simulink model "SCo2"  (Simulink 8.5)
settings: Solver=ode23tb  SolverMode=SingleTasking  StartTime=0.0  StopTime=0.1  MaxStep=2e-4  RelTol=1e-3  AbsTol=1e-6
libraries: powerlib x100, powerlib_extras x21
(part 1 of 2)
settings Model: Creator=azadpour  LastModifiedBy=PC  ExtModeTrigMode=oneshot  ExtModeArmWhenConnect=off
settings DataIOCC: LimitDataPoints=off
settings OptimizationCC: BlockReduction=off  BooleanDataType=off  ExpressionDepthLimit=128  InitFltsAndDblsToZero=on
settings DebuggingCC: SaveWithParameterizedLinksMsg=none  SignalResolutionControl=TryResolveAllWithWarning  MultiTaskDSMMsg=warning  MultiTaskCondExecSysMsg=none  FcnCallInpInsideContextMsg=UseLocalSettings  StateNameClashWarn=none
settings HardwareCC: TargetUnknown=on
settings GRTTargetCC: TargetFcnLib=ansi_tfl_tmw.mat

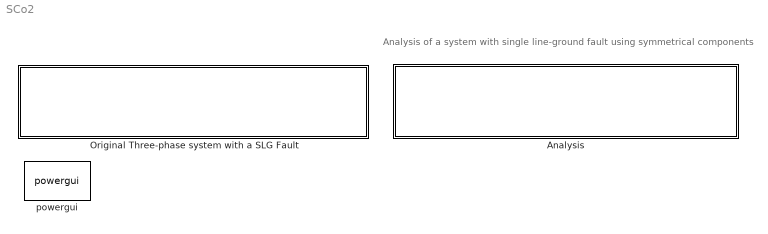
== system SCo2 ==
  note: Analysis of a system with single line-ground fault using symmetrical components
  Analysis : Subsystem
      mask init:
      | get_param('SCo2/Analysis/Fault Connection in Symmetrical Components','Name');
      mask Display: disp('Analysis of the system using Sequence Networks');
  Original Three-phase system with a SLG Fault : Subsystem
      mask Display: disp('Original Three-phase system with a SLG Fault')
  powergui : powerlib/powergui  Priority=1  SimulationMode=Continuous  SolverType=Tustin/Backward Euler (TBE)  SampleTime=50e-6  frequency=60  SPID=off  DisableSnubberDevices=off  DisableRonSwitches=off  DisableVfSwitches=off  SwTol=0  DisplayEquations=off  Interpol=off  methode=off  Ts=100  FunctionMessages=off  echomessages=off  HookPort=off  EnableUseOfTLC=off  x0status=blocks  frequencyindice=60  Pbase=100e6  ErrMax=1e-4  Iterations=50  UnitsV=kV  UnitsW=MW  buscounter=0  RestoreLinks=warning  ResistiveCurrentMeasurement=off  Frange=[0:2:500]  Ylog=off  Xlog=on  ShowGrid=off  save=off  variable=ZData  structure=0  ZoomFFT=off  StartTime=0.0  cycles=1  DisplayStyle=1  fundamental=60  FreqAxis=off  MaxFrequency=1000  frequencyindicesteady=1  RmsSteady=1  display=off

== system SCo2/Analysis ==
  note: Analysis using symmetrical networks
  Connected Symmetrical Networks : Subsystem
      mask Display: disp('Connected\n Sequence\n Networks')
  Fault Connection in Symmetrical Components : Subsystem
      mask Display: disp('Fault connection\n in\n symmetrical components')
  Negative Sequence Network : Subsystem
      mask Display: disp('Negative sequence network')
  Positive Sequence Network : Subsystem
      mask Display: disp('Positive sequence network')
  Zero Sequence Network : Subsystem
      mask Display: disp('Zero sequence network')

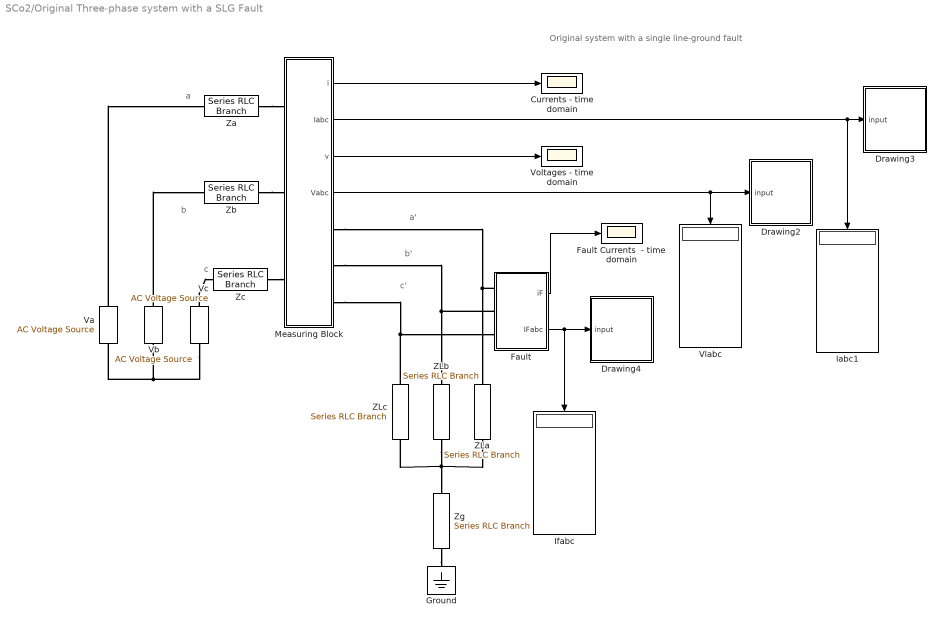
== system SCo2/Original Three-phase system with a SLG Fault ==
  note: a
  note: a'
  note: b
  note: b'
  note: c'
  note: c
  note: Original system with a single line-ground fault
  Currents - time domain : Scope
      settings: TickLabels=on
  Drawing2 : Subsystem  mask(ABC and 012 Phasor Display){Bactive=off}
      mask prompts: Bactive "Block active"
      mask init:
      | global count;
      | count=0;
      mask Display: disp('Display \nabc \nand \n012\nphasors');
  Drawing3 : Subsystem  mask(ABC and 012 Phasor Display){Bactive=off}
      mask prompts: Bactive "Block active"
      mask init:
      | global count;
      | count=0;
      mask Display: disp('Display \nabc \nand \n012\nphasors');
  Drawing4 : Subsystem  mask(ABC and 012 Phasor Display){Bactive=off}
      mask prompts: Bactive "Block active"
      mask init:
      | global count;
      | count=0;
      mask Display: disp('Display \nabc \nand \n012\nphasors');
  Fault : Subsystem
  Fault Currents  - time domain : Scope
      settings: TickLabels=on
  Ground : powerlib/Elements/Ground  LConnTagsString=a
  Iabc1 : Display
  Ifabc : Display
  Measuring Block : Subsystem
  Va : powerlib/Electrical Sources/AC Voltage Source  Amplitude=1  Phase=0  Frequency=60  SampleTime=0  Measurements=None
  Vb : powerlib/Electrical Sources/AC Voltage Source  Amplitude=1  Phase=-120  Frequency=60  SampleTime=0  Measurements=None
  Vc : powerlib/Electrical Sources/AC Voltage Source  Amplitude=1  Phase=120  Frequency=60  SampleTime=0  Measurements=None
  Vlabc : Display
  Voltages - time domain : Scope
      settings: TickLabels=on
  ZLa : powerlib/Elements/Series RLC Branch  LConnTagsString=__new0  RConnTagsString=__new0  BranchType=RL  Resistance=0.1736  Inductance=0.9848/(2*pi*60)  SetiL0=off  InitialCurrent=0  Capacitance=1.0  Setx0=off  InitialVoltage=0  Measurements=None
  ZLb : powerlib/Elements/Series RLC Branch  LConnTagsString=__new0  RConnTagsString=__new0  BranchType=RL  Resistance=0.1736  Inductance=0.9848/(2*pi*60)  SetiL0=off  InitialCurrent=0  Capacitance=1.0  Setx0=off  InitialVoltage=0  Measurements=None
  ZLc : powerlib/Elements/Series RLC Branch  LConnTagsString=__new0  RConnTagsString=__new0  BranchType=RL  Resistance=0.1736  Inductance=0.9848/(2*pi*60)  SetiL0=off  InitialCurrent=0  Capacitance=1.0  Setx0=off  InitialVoltage=0  Measurements=None
  Za : powerlib/Elements/Series RLC Branch  LConnTagsString=__new0  RConnTagsString=__new0  BranchType=RL  Resistance=0.0347  Inductance=0.1970/(2*pi*60)  SetiL0=off  InitialCurrent=0  Capacitance=1.0  Setx0=off  InitialVoltage=0  Measurements=None
  Zb : powerlib/Elements/Series RLC Branch  LConnTagsString=__new0  RConnTagsString=__new0  BranchType=RL  Resistance=0.0347  Inductance=0.1970/(2*pi*60)  SetiL0=off  InitialCurrent=0  Capacitance=1.0  Setx0=off  InitialVoltage=0  Measurements=None
  Zc : powerlib/Elements/Series RLC Branch  LConnTagsString=__new0  RConnTagsString=__new0  BranchType=RL  Resistance=0.0347  Inductance=0.1970/(2*pi*60)  SetiL0=off  InitialCurrent=0  Capacitance=1.0  Setx0=off  InitialVoltage=0  Measurements=None
  Zg : powerlib/Elements/Series RLC Branch  LConnTagsString=__new0  RConnTagsString=__new0  BranchType=RL  Resistance=0.0695  Inductance=0.3939/(2*pi*60)  SetiL0=off  InitialCurrent=0  Capacitance=1.0  Setx0=off  InitialVoltage=0  Measurements=None
  wires:
  Fault/1(iF) -> Fault Currents  - time domain/1
  Fault/2(IFabc) -> Drawing4/1(input), Ifabc/1
  Measuring Block/1(i) -> Currents - time domain/1
  Measuring Block/4(Vabc) -> Drawing2/1(input), Vlabc/1
  Measuring Block/3(v) -> Voltages - time domain/1
  Measuring Block/2(Iabc) -> Drawing3/1(input), Iabc1/1
  connections:
  Vc/LConn1 -- Va/LConn1 -- Vb/LConn1
  Va/RConn1 -- Za/LConn1
  Vc/RConn1 -- Zc/LConn1
  Za/RConn1 -- Measuring Block/LConn1
  Zc/RConn1 -- Measuring Block/LConn3
  Vb/RConn1 -- Zb/LConn1
  Zb/RConn1 -- Measuring Block/LConn2
  ZLc/LConn1 -- Fault/LConn3 -- Measuring Block/RConn3
  Fault/LConn2 -- ZLb/LConn1 -- Measuring Block/RConn2
  Fault/LConn1 -- ZLa/LConn1 -- Measuring Block/RConn1
  ZLa/RConn1 -- ZLc/RConn1 -- ZLb/RConn1 -- Zg/LConn1
  Zg/RConn1 -- Ground/LConn1

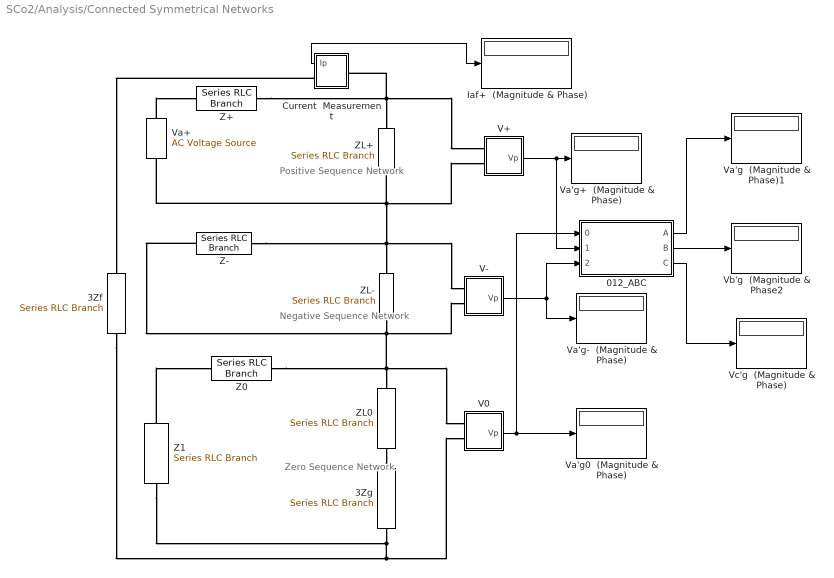
== system SCo2/Analysis/Connected Symmetrical Networks ==
  note: Positive Sequence Network
  note: Negative Sequence Network
  note: Zero Sequence Network
  012_ABC : Subsystem
      mask init:
      | a=cos(120*pi/180)+i*sin(120*pi/180);
      | A=[1 1 1; 1 a^2 a; 1 a a^2];
      mask Display: disp('012_ABC');
  3Zf : powerlib/Elements/Series RLC Branch  LConnTagsString=__new0  RConnTagsString=__new0  BranchType=RL  Resistance=3*0.0174  Inductance=3*0.0985/(2*pi*60)  SetiL0=off  InitialCurrent=0  Capacitance=1.0  Setx0=off  InitialVoltage=0  Measurements=None
  3Zg : powerlib/Elements/Series RLC Branch  LConnTagsString=__new0  RConnTagsString=__new0  BranchType=RL  Resistance=3*0.0695  Inductance=3*0.3939/(2*pi*60)  SetiL0=off  InitialCurrent=0  Capacitance=1.0  Setx0=off  InitialVoltage=0  Measurements=None
  Current  Measurement : Subsystem
  Iaf+  (Magnitude & Phase) : Display
  V+ : Subsystem
  V- : Subsystem
  V0 : Subsystem
  Va'g  (Magnitude & Phase)1 : Display
  Va'g+  (Magnitude & Phase) : Display
  Va'g-  (Magnitude & Phase) : Display
  Va'g0  (Magnitude & Phase) : Display
  Va+ : powerlib/Electrical Sources/AC Voltage Source  Amplitude=1  Phase=0  Frequency=60  SampleTime=0  Measurements=None
  Vb'g  (Magnitude & Phase2 : Display
  Vc'g  (Magnitude & Phase) : Display
  Z+ : powerlib/Elements/Series RLC Branch  LConnTagsString=__new0  RConnTagsString=__new0  BranchType=RL  Resistance=0.0347  Inductance=0.1970/(2*pi*60)  SetiL0=off  InitialCurrent=0  Capacitance=1.0  Setx0=off  InitialVoltage=0  Measurements=None
  Z- : powerlib/Elements/Series RLC Branch  LConnTagsString=__new0  RConnTagsString=__new0  BranchType=RL  Resistance=0.0347  Inductance=0.1970/(2*pi*60)  SetiL0=off  InitialCurrent=0  Capacitance=1.0  Setx0=off  InitialVoltage=0  Measurements=None
  Z0 : powerlib/Elements/Series RLC Branch  LConnTagsString=__new0  RConnTagsString=__new0  BranchType=RL  Resistance=0.0347  Inductance=0.1970/(2*pi*60)  SetiL0=off  InitialCurrent=0  Capacitance=1.0  Setx0=off  InitialVoltage=0  Measurements=None
  Z1 : powerlib/Elements/Series RLC Branch  LConnTagsString=__new0  RConnTagsString=__new0  BranchType=Open circuit  Resistance=1  Inductance=1.0  SetiL0=off  InitialCurrent=0  Capacitance=1.0  Setx0=off  InitialVoltage=0  Measurements=None
  ZL+ : powerlib/Elements/Series RLC Branch  LConnTagsString=__new0  RConnTagsString=__new0  BranchType=RL  Resistance=0.1736  Inductance=0.9848/(2*pi*60)  SetiL0=off  InitialCurrent=0  Capacitance=1.0  Setx0=off  InitialVoltage=0  Measurements=None
  ZL- : powerlib/Elements/Series RLC Branch  LConnTagsString=__new0  RConnTagsString=__new0  BranchType=RL  Resistance=0.1736  Inductance=0.9848/(2*pi*60)  SetiL0=off  InitialCurrent=0  Capacitance=1.0  Setx0=off  InitialVoltage=0  Measurements=None
  ZL0 : powerlib/Elements/Series RLC Branch  LConnTagsString=__new0  RConnTagsString=__new0  BranchType=RL  Resistance=0.1736  Inductance=0.9848/(2*pi*60)  SetiL0=off  InitialCurrent=0  Capacitance=1.0  Setx0=off  InitialVoltage=0  Measurements=None
  wires:
  Current  Measurement/1(Ip) -> Iaf+  (Magnitude & Phase)/1
  012_ABC/1(A) -> Va'g  (Magnitude & Phase)1/1
  012_ABC/2(B) -> Vb'g  (Magnitude & Phase2/1
  012_ABC/3(C) -> Vc'g  (Magnitude & Phase)/1
  V0/1(Vp) -> Va'g0  (Magnitude & Phase)/1, 012_ABC/1(0)
  V+/1(Vp) -> Va'g+  (Magnitude & Phase)/1, 012_ABC/2(1)
  V-/1(Vp) -> Va'g-  (Magnitude & Phase)/1, 012_ABC/3(2)
  connections:
  Z1/RConn1 -- 3Zf/RConn1 -- V0/LConn2 -- 3Zg/RConn1
  Va+/RConn1 -- Z+/LConn1
  V-/LConn1 -- ZL-/LConn1 -- Z-/RConn1 -- Va+/LConn1 -- V+/LConn2 -- ZL+/RConn1
  Z+/RConn1 -- V+/LConn1 -- ZL+/LConn1 -- Current  Measurement/LConn1
  Current  Measurement/RConn1 -- 3Zf/LConn1
  Z0/RConn1 -- V-/LConn2 -- ZL-/RConn1 -- Z-/LConn1 -- ZL0/LConn1 -- V0/LConn1
  Z1/LConn1 -- Z0/LConn1
  ZL0/RConn1 -- 3Zg/LConn1

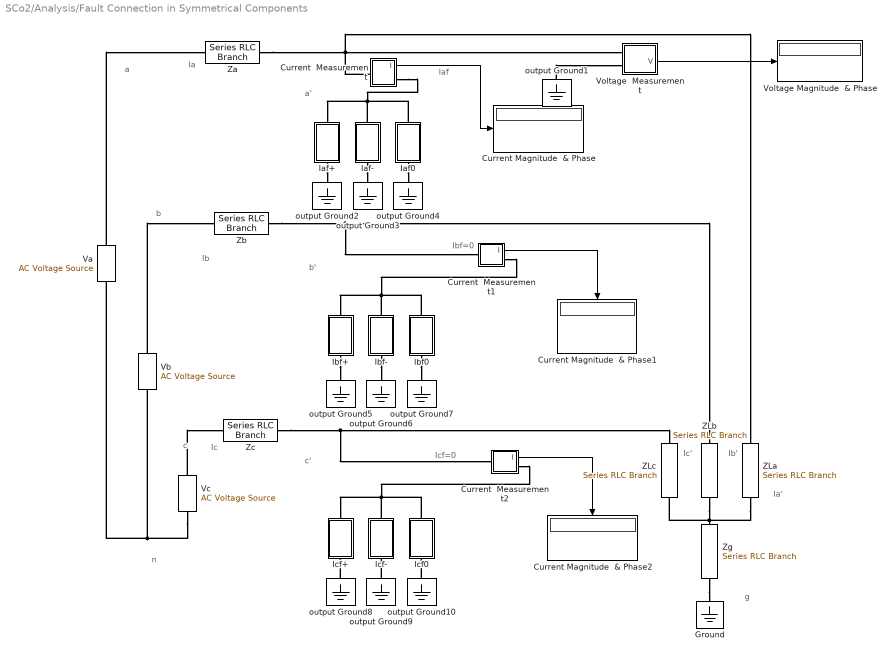
== system SCo2/Analysis/Fault Connection in Symmetrical Components ==
  note: Ibf=0
  note: Icf=0
  note: Ia
  note: Ib
  note: Ic
  note: Ia'
  note: Ib'
  note: Ic'
  note: a
  note: b
  note: c
  note: c'
  note: b'
  note: a'
  note: Iaf
  note: g
  note: n
  Current  Measurement : Subsystem
  Current  Measurement1 : Subsystem
  Current  Measurement2 : Subsystem
  Current Magnitude  & Phase : Display
  Current Magnitude  & Phase1 : Display
  Current Magnitude  & Phase2 : Display
  Ground : powerlib/Elements/Ground  LConnTagsString=a
  Iaf+ : Subsystem  mask{A=-0.8823/3, P=-80, F=60}
      mask prompts: A "Peak amplitude(A)"; P "Phase (deg)"; F "Freqiuency"
      mask Display: plot(-50,-35,50,50-15,[0,9,18,24,29,30,29,24,18,9,0,-9,-18,-24,-29,-30,-29,-24,-18,-9,0],[30,29,24,18,9,0,-9,-18,-24,-29,-30,-29,-24,-18,-9,0,9,18,24,29,30],[-20 5 5 20 5 5],[2 2 12 2 -8 2],[-50 -30],[0 0],[50,30],[0 0],[45 35 40 40 40],[15 15 15 20 10]);
  Iaf- : Subsystem  mask{A=-0.8823/3, P=-80, F=60}
      mask prompts: A "Peak amplitude(A)"; P "Phase (deg)"; F "Freqiuency"
      mask Display: plot(-50,-35,50,50-15,[0,9,18,24,29,30,29,24,18,9,0,-9,-18,-24,-29,-30,-29,-24,-18,-9,0],[30,29,24,18,9,0,-9,-18,-24,-29,-30,-29,-24,-18,-9,0,9,18,24,29,30],[-20 5 5 20 5 5],[2 2 12 2 -8 2],[-50 -30],[0 0],[50,30],[0 0],[45 35 40 40 40],[15 15 15 20 10]);
  Iaf0 : Subsystem  mask{A=-0.8823/3, P=-80, F=60}
      mask prompts: A "Peak amplitude(A)"; P "Phase (deg)"; F "Freqiuency"
      mask Display: plot(-50,-35,50,50-15,[0,9,18,24,29,30,29,24,18,9,0,-9,-18,-24,-29,-30,-29,-24,-18,-9,0],[30,29,24,18,9,0,-9,-18,-24,-29,-30,-29,-24,-18,-9,0,9,18,24,29,30],[-20 5 5 20 5 5],[2 2 12 2 -8 2],[-50 -30],[0 0],[50,30],[0 0],[45 35 40 40 40],[15 15 15 20 10]);
  Ibf+ : Subsystem  mask{A=-0.8823/3, P=-80-120, F=60}
      mask prompts: A "Peak amplitude(A)"; P "Phase (deg)"; F "Freqiuency"
      mask Display: plot(-50,-35,50,50-15,[0,9,18,24,29,30,29,24,18,9,0,-9,-18,-24,-29,-30,-29,-24,-18,-9,0],[30,29,24,18,9,0,-9,-18,-24,-29,-30,-29,-24,-18,-9,0,9,18,24,29,30],[-20 5 5 20 5 5],[2 2 12 2 -8 2],[-50 -30],[0 0],[50,30],[0 0],[45 35 40 40 40],[15 15 15 20 10]);
  Ibf- : Subsystem  mask{A=-0.8823/3, P=-80+120, F=60}
      mask prompts: A "Peak amplitude(A)"; P "Phase (deg)"; F "Freqiuency"
      mask Display: plot(-50,-35,50,50-15,[0,9,18,24,29,30,29,24,18,9,0,-9,-18,-24,-29,-30,-29,-24,-18,-9,0],[30,29,24,18,9,0,-9,-18,-24,-29,-30,-29,-24,-18,-9,0,9,18,24,29,30],[-20 5 5 20 5 5],[2 2 12 2 -8 2],[-50 -30],[0 0],[50,30],[0 0],[45 35 40 40 40],[15 15 15 20 10]);
  Ibf0 : Subsystem  mask{A=-0.8823/3, P=-80, F=60}
      mask prompts: A "Peak amplitude(A)"; P "Phase (deg)"; F "Freqiuency"
      mask Display: plot(-50,-35,50,50-15,[0,9,18,24,29,30,29,24,18,9,0,-9,-18,-24,-29,-30,-29,-24,-18,-9,0],[30,29,24,18,9,0,-9,-18,-24,-29,-30,-29,-24,-18,-9,0,9,18,24,29,30],[-20 5 5 20 5 5],[2 2 12 2 -8 2],[-50 -30],[0 0],[50,30],[0 0],[45 35 40 40 40],[15 15 15 20 10]);
  Icf+ : Subsystem  mask{A=-0.8823/3, P=-80+120, F=60}
      mask prompts: A "Peak amplitude(A)"; P "Phase (deg)"; F "Freqiuency"
      mask Display: plot(-50,-35,50,50-15,[0,9,18,24,29,30,29,24,18,9,0,-9,-18,-24,-29,-30,-29,-24,-18,-9,0],[30,29,24,18,9,0,-9,-18,-24,-29,-30,-29,-24,-18,-9,0,9,18,24,29,30],[-20 5 5 20 5 5],[2 2 12 2 -8 2],[-50 -30],[0 0],[50,30],[0 0],[45 35 40 40 40],[15 15 15 20 10]);
  Icf- : Subsystem  mask{A=-0.8823/3, P=-80-120, F=60}
      mask prompts: A "Peak amplitude(A)"; P "Phase (deg)"; F "Freqiuency"
      mask Display: plot(-50,-35,50,50-15,[0,9,18,24,29,30,29,24,18,9,0,-9,-18,-24,-29,-30,-29,-24,-18,-9,0],[30,29,24,18,9,0,-9,-18,-24,-29,-30,-29,-24,-18,-9,0,9,18,24,29,30],[-20 5 5 20 5 5],[2 2 12 2 -8 2],[-50 -30],[0 0],[50,30],[0 0],[45 35 40 40 40],[15 15 15 20 10]);
  Icf0 : Subsystem  mask{A=-0.8823/3, P=-80, F=60}
      mask prompts: A "Peak amplitude(A)"; P "Phase (deg)"; F "Freqiuency"
      mask Display: plot(-50,-35,50,50-15,[0,9,18,24,29,30,29,24,18,9,0,-9,-18,-24,-29,-30,-29,-24,-18,-9,0],[30,29,24,18,9,0,-9,-18,-24,-29,-30,-29,-24,-18,-9,0,9,18,24,29,30],[-20 5 5 20 5 5],[2 2 12 2 -8 2],[-50 -30],[0 0],[50,30],[0 0],[45 35 40 40 40],[15 15 15 20 10]);
  Va : powerlib/Electrical Sources/AC Voltage Source  Amplitude=1  Phase=0  Frequency=60  SampleTime=0  Measurements=None
  Vb : powerlib/Electrical Sources/AC Voltage Source  Amplitude=1  Phase=-120  Frequency=60  SampleTime=0  Measurements=None
  Vc : powerlib/Electrical Sources/AC Voltage Source  Amplitude=1  Phase=120  Frequency=60  SampleTime=0  Measurements=None
  Voltage  Measurement : Subsystem
  Voltage Magnitude  & Phase : Display
  ZLa : powerlib/Elements/Series RLC Branch  LConnTagsString=__new0  RConnTagsString=__new0  BranchType=RL  Resistance=0.1736  Inductance=0.9848/(2*pi*60)  SetiL0=off  InitialCurrent=0  Capacitance=1.0  Setx0=off  InitialVoltage=0  Measurements=None
  ZLb : powerlib/Elements/Series RLC Branch  LConnTagsString=__new0  RConnTagsString=__new0  BranchType=RL  Resistance=0.1736  Inductance=0.9848/(2*pi*60)  SetiL0=off  InitialCurrent=0  Capacitance=1.0  Setx0=off  InitialVoltage=0  Measurements=None
  ZLc : powerlib/Elements/Series RLC Branch  LConnTagsString=__new0  RConnTagsString=__new0  BranchType=RL  Resistance=0.1736  Inductance=0.9848/(2*pi*60)  SetiL0=off  InitialCurrent=0  Capacitance=1.0  Setx0=off  InitialVoltage=0  Measurements=None
  Za : powerlib/Elements/Series RLC Branch  LConnTagsString=__new0  RConnTagsString=__new0  BranchType=RL  Resistance=0.0347  Inductance=0.1970/(2*pi*60)  SetiL0=off  InitialCurrent=0  Capacitance=1.0  Setx0=off  InitialVoltage=0  Measurements=None
  Zb : powerlib/Elements/Series RLC Branch  LConnTagsString=__new0  RConnTagsString=__new0  BranchType=RL  Resistance=0.0347  Inductance=0.1970/(2*pi*60)  SetiL0=off  InitialCurrent=0  Capacitance=1.0  Setx0=off  InitialVoltage=0  Measurements=None
  Zc : powerlib/Elements/Series RLC Branch  LConnTagsString=__new0  RConnTagsString=__new0  BranchType=RL  Resistance=0.0347  Inductance=0.1970/(2*pi*60)  SetiL0=off  InitialCurrent=0  Capacitance=1.0  Setx0=off  InitialVoltage=0  Measurements=None
  Zg : powerlib/Elements/Series RLC Branch  LConnTagsString=__new0  RConnTagsString=__new0  BranchType=RL  Resistance=0.0695  Inductance=0.3939/(2*pi*60)  SetiL0=off  InitialCurrent=0  Capacitance=1.0  Setx0=off  InitialVoltage=0  Measurements=None
  output Ground{1..10} (10 alike) : powerlib/Elements/Ground  LConnTagsString=a
  wires:
  Current  Measurement/1(I) -> Current Magnitude  & Phase/1
  Current  Measurement2/1(I) -> Current Magnitude  & Phase2/1
  Voltage  Measurement/1(V) -> Voltage Magnitude  & Phase/1
  Current  Measurement1/1(I) -> Current Magnitude  & Phase1/1
  connections:
  Va/RConn1 -- Za/LConn1
  output Ground1/LConn1 -- Voltage  Measurement/LConn2
  Vb/RConn1 -- Zb/LConn1
  Vc/RConn1 -- Zc/LConn1
  Zc/RConn1 -- ZLc/LConn1 -- Current  Measurement2/LConn1
  Zg/RConn1 -- Ground/LConn1
  Ibf+/LConn1 -- output Ground5/LConn1
  Ibf-/LConn1 -- output Ground6/LConn1
  Ibf0/LConn1 -- output Ground7/LConn1
  Ibf0/RConn1 -- Ibf+/RConn1 -- Ibf-/RConn1 -- Current  Measurement1/RConn1
  output Ground8/LConn1 -- Icf+/LConn1
  output Ground9/LConn1 -- Icf-/LConn1
  output Ground10/LConn1 -- Icf0/LConn1
  Icf0/RConn1 -- Icf+/RConn1 -- Icf-/RConn1 -- Current  Measurement2/RConn1
  ZLa/RConn1 -- ZLb/RConn1 -- Zg/LConn1 -- ZLc/RConn1
  Iaf0/RConn1 -- Iaf+/RConn1 -- Iaf-/RConn1 -- Current  Measurement/RConn1
  Iaf+/LConn1 -- output Ground2/LConn1
  Iaf-/LConn1 -- output Ground3/LConn1
  Iaf0/LConn1 -- output Ground4/LConn1
  Vc/LConn1 -- Va/LConn1 -- Vb/LConn1
  Current  Measurement/LConn1 -- Voltage  Measurement/LConn1 -- ZLa/LConn1 -- Za/RConn1
  Zb/RConn1 -- ZLb/LConn1 -- Current  Measurement1/LConn1

== system SCo2/Analysis/Negative Sequence Network ==
  Current  Measurement : Subsystem
  Iaf- : Subsystem  mask{A=-0.8823/3, P=-80, F=60}
      mask prompts: A "Peak amplitude(A)"; P "Phase (deg)"; F "Freqiuency"
      mask Display: plot(-50,-35,50,50-15,[0,9,18,24,29,30,29,24,18,9,0,-9,-18,-24,-29,-30,-29,-24,-18,-9,0],[30,29,24,18,9,0,-9,-18,-24,-29,-30,-29,-24,-18,-9,0,9,18,24,29,30],[-20 5 5 20 5 5],[2 2 12 2 -8 2],[-50 -30],[0 0],[50,30],[0 0],[45 35 40 40 40],[15 15 15 20 10]);
  Iaf- (Magnitude & Phase) : Display
  V- : Subsystem
  Va'g- (Magnitude & Phase) : Display
  ZLa : powerlib/Elements/Series RLC Branch  LConnTagsString=__new0  RConnTagsString=__new0  BranchType=RL  Resistance=0.1736  Inductance=0.9848/(2*pi*60)  SetiL0=off  InitialCurrent=0  Capacitance=1.0  Setx0=off  InitialVoltage=0  Measurements=None
  Za : powerlib/Elements/Series RLC Branch  LConnTagsString=__new0  RConnTagsString=__new0  BranchType=RL  Resistance=0.0347  Inductance=0.1970/(2*pi*60)  SetiL0=off  InitialCurrent=0  Capacitance=1.0  Setx0=off  InitialVoltage=0  Measurements=None
  wires:
  Current  Measurement/1(I) -> Iaf- (Magnitude & Phase)/1
  V-/1(V) -> Va'g- (Magnitude & Phase)/1
  connections:
  Za/RConn1 -- ZLa/LConn1 -- V-/LConn1 -- Current  Measurement/LConn1
  ZLa/RConn1 -- V-/LConn2 -- Za/LConn1 -- Iaf-/LConn1
  Current  Measurement/RConn1 -- Iaf-/RConn1

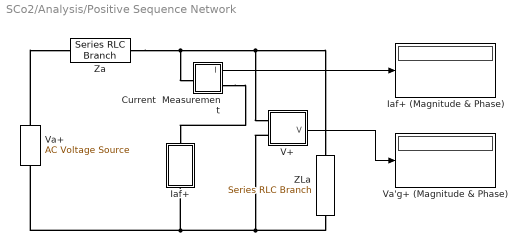
== system SCo2/Analysis/Positive Sequence Network ==
  Current  Measurement : Subsystem
  Iaf+ : Subsystem  mask{A=-0.8823/3, P=-80, F=60}
      mask prompts: A "Peak amplitude(A)"; P "Phase (deg)"; F "Freqiuency"
      mask Display: plot(-50,-35,50,50-15,[0,9,18,24,29,30,29,24,18,9,0,-9,-18,-24,-29,-30,-29,-24,-18,-9,0],[30,29,24,18,9,0,-9,-18,-24,-29,-30,-29,-24,-18,-9,0,9,18,24,29,30],[-20 5 5 20 5 5],[2 2 12 2 -8 2],[-50 -30],[0 0],[50,30],[0 0],[45 35 40 40 40],[15 15 15 20 10]);
  Iaf+ (Magnitude & Phase) : Display
  V+ : Subsystem
  Va'g+ (Magnitude & Phase) : Display
  Va+ : powerlib/Electrical Sources/AC Voltage Source  Amplitude=1  Phase=0  Frequency=60  SampleTime=0  Measurements=None
  ZLa : powerlib/Elements/Series RLC Branch  LConnTagsString=__new0  RConnTagsString=__new0  BranchType=RL  Resistance=0.1736  Inductance=0.9848/(2*pi*60)  SetiL0=off  InitialCurrent=0  Capacitance=1.0  Setx0=off  InitialVoltage=0  Measurements=None
  Za : powerlib/Elements/Series RLC Branch  LConnTagsString=__new0  RConnTagsString=__new0  BranchType=RL  Resistance=0.0347  Inductance=0.1970/(2*pi*60)  SetiL0=off  InitialCurrent=0  Capacitance=1.0  Setx0=off  InitialVoltage=0  Measurements=None
  wires:
  Current  Measurement/1(I) -> Iaf+ (Magnitude & Phase)/1
  V+/1(V) -> Va'g+ (Magnitude & Phase)/1
  connections:
  Va+/RConn1 -- Za/LConn1
  Za/RConn1 -- Current  Measurement/LConn1 -- ZLa/LConn1 -- V+/LConn1
  V+/LConn2 -- ZLa/RConn1 -- Iaf+/LConn1 -- Va+/LConn1
  Current  Measurement/RConn1 -- Iaf+/RConn1

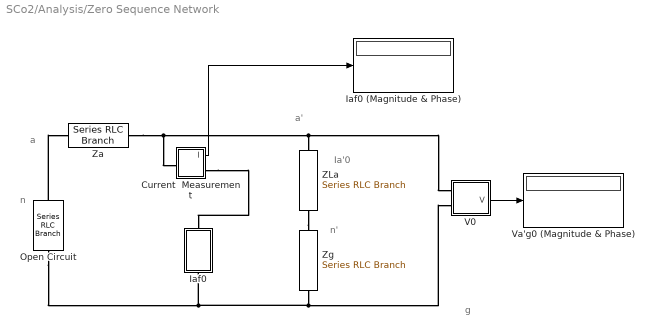
== system SCo2/Analysis/Zero Sequence Network ==
  note: n'
  note: n
  note: a
  note: a'
  note: g
  note: Ia'0
  Current  Measurement : Subsystem
  Iaf0 : Subsystem  mask{A=-0.8823/3, P=-80, F=60}
      mask prompts: A "Peak amplitude(A)"; P "Phase (deg)"; F "Freqiuency"
      mask Display: plot(-50,-35,50,50-15,[0,9,18,24,29,30,29,24,18,9,0,-9,-18,-24,-29,-30,-29,-24,-18,-9,0],[30,29,24,18,9,0,-9,-18,-24,-29,-30,-29,-24,-18,-9,0,9,18,24,29,30],[-20 5 5 20 5 5],[2 2 12 2 -8 2],[-50 -30],[0 0],[50,30],[0 0],[45 35 40 40 40],[15 15 15 20 10]);
  Iaf0 (Magnitude & Phase) : Display
  Open Circuit : powerlib/Elements/Series RLC Branch  LConnTagsString=__new0  RConnTagsString=__new0  BranchType=Open circuit  Resistance=1  Inductance=1e-3  SetiL0=off  InitialCurrent=0  Capacitance=1e-6  Setx0=off  InitialVoltage=0  Measurements=None
  V0 : Subsystem
  Va'g0 (Magnitude & Phase) : Display
  ZLa : powerlib/Elements/Series RLC Branch  LConnTagsString=__new0  RConnTagsString=__new0  BranchType=RL  Resistance=0.1736  Inductance=0.9848/(2*pi*60)  SetiL0=off  InitialCurrent=0  Capacitance=1.0  Setx0=off  InitialVoltage=0  Measurements=None
  Za : powerlib/Elements/Series RLC Branch  LConnTagsString=__new0  RConnTagsString=__new0  BranchType=RL  Resistance=0.0347  Inductance=0.1970/(2*pi*60)  SetiL0=off  InitialCurrent=0  Capacitance=1.0  Setx0=off  InitialVoltage=0  Measurements=None
  Zg : powerlib/Elements/Series RLC Branch  LConnTagsString=__new0  RConnTagsString=__new0  BranchType=RL  Resistance=3*0.0695  Inductance=3*0.3939/(2*pi*60)  SetiL0=off  InitialCurrent=0  Capacitance=1.0  Setx0=off  InitialVoltage=0  Measurements=None
  wires:
  Current  Measurement/1(I) -> Iaf0 (Magnitude & Phase)/1
  V0/1(V) -> Va'g0 (Magnitude & Phase)/1
  connections:
  Za/RConn1 -- ZLa/LConn1 -- V0/LConn1 -- Current  Measurement/LConn1
  Zg/RConn1 -- V0/LConn2 -- Open Circuit/RConn1 -- Iaf0/LConn1
  ZLa/RConn1 -- Zg/LConn1
  Current  Measurement/RConn1 -- Iaf0/RConn1
  Open Circuit/LConn1 -- Za/LConn1

== system SCo2/Original Three-phase system with a SLG Fault/Drawing2 ==
  input : Inport
  S-Function : S-Function  FunctionName=phdraw1c  Parameters=Bactive
  wires:
  input/1 -> S-Function/1

== system SCo2/Original Three-phase system with a SLG Fault/Drawing3 ==
  input : Inport
  S-Function : S-Function  FunctionName=phdraw1c  Parameters=Bactive
  wires:
  input/1 -> S-Function/1

== system SCo2/Original Three-phase system with a SLG Fault/Drawing4 ==
  input : Inport
  S-Function : S-Function  FunctionName=phdraw1c  Parameters=Bactive
  wires:
  input/1 -> S-Function/1

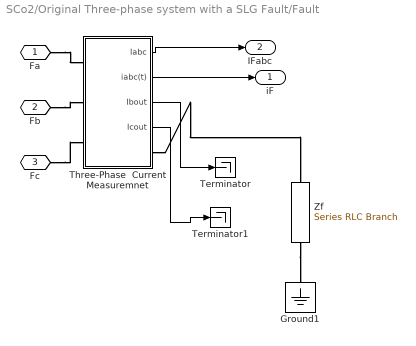
== system SCo2/Original Three-phase system with a SLG Fault/Fault ==
  Ground1 : powerlib/Elements/Ground  LConnTagsString=a
  Terminator : Terminator
  Terminator1 : Terminator
  Three-Phase  Current Measuremnet : Subsystem
  Zf : powerlib/Elements/Series RLC Branch  LConnTagsString=__new0  RConnTagsString=__new0  BranchType=RL  Resistance=0.0174  Inductance=0.0985/(2*pi*60)  SetiL0=off  InitialCurrent=0  Capacitance=1.0  Setx0=off  InitialVoltage=0  Measurements=None
  Fa : PMIOPort  Port=1  Side=Left
  Fb : PMIOPort  Port=2  Side=Left
  Fc : PMIOPort  Port=3  Side=Left
  iF : Outport
  IFabc : Outport  Port=2
  wires:
  Three-Phase  Current Measuremnet/1(Iabc) -> IFabc/1
  Three-Phase  Current Measuremnet/3(Ibout) -> Terminator/1
  Three-Phase  Current Measuremnet/4(Icout) -> Terminator1/1
  Three-Phase  Current Measuremnet/2(iabc(t)) -> iF/1
  connections:
  Three-Phase  Current Measuremnet/RConn1 -- Zf/LConn1
  Zf/RConn1 -- Ground1/LConn1
  Fb/RConn1 -- Three-Phase  Current Measuremnet/LConn2
  Fc/RConn1 -- Three-Phase  Current Measuremnet/LConn3
  Fa/RConn1 -- Three-Phase  Current Measuremnet/LConn1

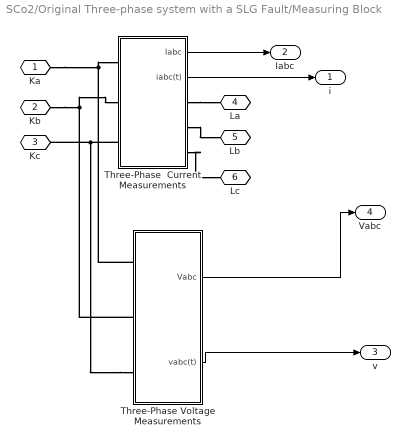
== system SCo2/Original Three-phase system with a SLG Fault/Measuring Block ==
  Three-Phase Voltage Measurements : Subsystem
  Three-Phase  Current Measurements : Subsystem
  Ka : PMIOPort  Port=1  Side=Left
  Kb : PMIOPort  Port=2  Side=Left
  Kc : PMIOPort  Port=3  Side=Left
  La : PMIOPort  Port=4  Side=Right
  Lb : PMIOPort  Port=5  Side=Right
  Lc : PMIOPort  Port=6  Side=Right
  i : Outport
  Iabc : Outport  Port=2
  v : Outport  Port=3
  Vabc : Outport  Port=4
  wires:
  Three-Phase  Current Measurements/1(Iabc) -> Iabc/1
  Three-Phase Voltage Measurements/1(Vabc) -> Vabc/1
  Three-Phase  Current Measurements/2(iabc(t)) -> i/1
  Three-Phase Voltage Measurements/2(vabc(t)) -> v/1
  connections:
  Three-Phase Voltage Measurements/LConn1 -- Ka/RConn1 -- Three-Phase  Current Measurements/LConn1
  Three-Phase Voltage Measurements/LConn2 -- Kb/RConn1 -- Three-Phase  Current Measurements/LConn2
  Three-Phase Voltage Measurements/LConn3 -- Kc/RConn1 -- Three-Phase  Current Measurements/LConn3
  Three-Phase  Current Measurements/RConn3 -- Lc/RConn1
  Three-Phase  Current Measurements/RConn2 -- Lb/RConn1
  Three-Phase  Current Measurements/RConn1 -- La/RConn1

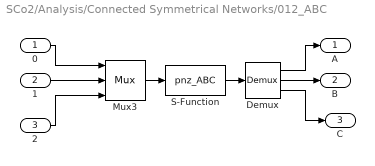
== system SCo2/Analysis/Connected Symmetrical Networks/012_ABC ==
  0 : Inport
  1 : Inport  Port=2
  2 : Inport  Port=3
  Demux : Demux  Outputs=3
  Mux3 : Mux  Inputs=3
  S-Function : S-Function  FunctionName=pnz_ABC  Parameters=A
  A : Outport  InitialOutput=0
  B : Outport  Port=2  InitialOutput=0
  C : Outport  Port=3  InitialOutput=0
  wires:
  Mux3/1 -> S-Function/1
  0/1 -> Mux3/1
  1/1 -> Mux3/2
  2/1 -> Mux3/3
  S-Function/1 -> Demux/1
  Demux/1 -> A/1
  Demux/2 -> B/1
  Demux/3 -> C/1

== system SCo2/Analysis/Connected Symmetrical Networks/Current  Measurement ==
  Current Measurement1 : powerlib/Measurements/Current Measurement  PhasorSimulation=off  OutputType=Magnitude  PSBequivalent=0
  Fourier1 : powerlib_extras/Measurements/Fourier  f1=60  n=1
  Mux1 : Mux  Inputs=2
  + : PMIOPort  Port=1  Side=Left
  - : PMIOPort  Port=2  Side=Right
  Ip : Outport  InitialOutput=0
  wires:
  Fourier1/2 -> Mux1/2
  Fourier1/1 -> Mux1/1
  Mux1/1 -> Ip/1
  Current Measurement1/1 -> Fourier1/1
  connections:
  +/RConn1 -- Current Measurement1/LConn1
  Current Measurement1/RConn1 -- -/RConn1

== system SCo2/Analysis/Connected Symmetrical Networks/V+ ==
  Fourier2 : powerlib_extras/Measurements/Fourier  f1=60  n=1
  Mux3 : Mux  Inputs=2
  Voltage Measurement1 : powerlib/Measurements/Voltage Measurement  PhasorSimulation=off  OutputType=Magnitude  PSBequivalent=0
  + : PMIOPort  Port=1  Side=Left
  - : PMIOPort  Port=2  Side=Left
  Vp : Outport  InitialOutput=0
  wires:
  Fourier2/1 -> Mux3/1
  Fourier2/2 -> Mux3/2
  Mux3/1 -> Vp/1
  Voltage Measurement1/1 -> Fourier2/1
  connections:
  +/RConn1 -- Voltage Measurement1/LConn1
  -/RConn1 -- Voltage Measurement1/LConn2

== system SCo2/Analysis/Connected Symmetrical Networks/V- ==
  Fourier2 : powerlib_extras/Measurements/Fourier  f1=60  n=1
  Mux3 : Mux  Inputs=2
  Voltage Measurement1 : powerlib/Measurements/Voltage Measurement  PhasorSimulation=off  OutputType=Magnitude  PSBequivalent=0
  + : PMIOPort  Port=1  Side=Left
  - : PMIOPort  Port=2  Side=Left
  Vp : Outport  InitialOutput=0
  wires:
  Fourier2/1 -> Mux3/1
  Fourier2/2 -> Mux3/2
  Mux3/1 -> Vp/1
  Voltage Measurement1/1 -> Fourier2/1
  connections:
  +/RConn1 -- Voltage Measurement1/LConn1
  -/RConn1 -- Voltage Measurement1/LConn2

== system SCo2/Analysis/Connected Symmetrical Networks/V0 ==
  Fourier2 : powerlib_extras/Measurements/Fourier  f1=60  n=1
  Mux3 : Mux  Inputs=2
  Voltage Measurement1 : powerlib/Measurements/Voltage Measurement  PhasorSimulation=off  OutputType=Magnitude  PSBequivalent=0
  + : PMIOPort  Port=1  Side=Left
  - : PMIOPort  Port=2  Side=Left
  Vp : Outport  InitialOutput=0
  wires:
  Mux3/1 -> Vp/1
  Fourier2/2 -> Mux3/2
  Fourier2/1 -> Mux3/1
  Voltage Measurement1/1 -> Fourier2/1
  connections:
  -/RConn1 -- Voltage Measurement1/LConn2
  +/RConn1 -- Voltage Measurement1/LConn1

== system SCo2/Analysis/Fault Connection in Symmetrical Components/Current  Measurement ==
  Current Magnitude  & Phase1 : Display
  Current Measurement1 : powerlib/Measurements/Current Measurement  PhasorSimulation=off  OutputType=Magnitude  PSBequivalent=0
  Fourier1 : powerlib_extras/Measurements/Fourier  f1=60  n=1
  Mux1 : Mux  Inputs=2
  + : PMIOPort  Port=1  Side=Left
  - : PMIOPort  Port=2  Side=Right
  I : Outport  InitialOutput=0
  wires:
  Fourier1/2 -> Mux1/2
  Fourier1/1 -> Mux1/1
  Mux1/1 -> I/1
  Current Measurement1/1 -> Fourier1/1, Current Magnitude  & Phase1/1
  connections:
  +/RConn1 -- Current Measurement1/LConn1
  Current Measurement1/RConn1 -- -/RConn1

== system SCo2/Analysis/Fault Connection in Symmetrical Components/Current  Measurement1 ==
  Current Magnitude  & Phase1 : Display
  Current Measurement1 : powerlib/Measurements/Current Measurement  PhasorSimulation=off  OutputType=Magnitude  PSBequivalent=0
  Fourier1 : powerlib_extras/Measurements/Fourier  f1=60  n=1
  Mux1 : Mux  Inputs=2
  + : PMIOPort  Port=1  Side=Left
  - : PMIOPort  Port=2  Side=Right
  I : Outport  InitialOutput=0
  wires:
  Mux1/1 -> I/1
  Fourier1/1 -> Mux1/1
  Fourier1/2 -> Mux1/2
  Current Measurement1/1 -> Current Magnitude  & Phase1/1, Fourier1/1
  connections:
  Current Measurement1/RConn1 -- -/RConn1
  +/RConn1 -- Current Measurement1/LConn1

== system SCo2/Analysis/Fault Connection in Symmetrical Components/Current  Measurement2 ==
  Current Magnitude  & Phase1 : Display
  Current Measurement1 : powerlib/Measurements/Current Measurement  PhasorSimulation=off  OutputType=Magnitude  PSBequivalent=0
  Fourier1 : powerlib_extras/Measurements/Fourier  f1=60  n=1
  Mux1 : Mux  Inputs=2
  + : PMIOPort  Port=1  Side=Left
  - : PMIOPort  Port=2  Side=Right
  I : Outport  InitialOutput=0
  wires:
  Fourier1/2 -> Mux1/2
  Fourier1/1 -> Mux1/1
  Mux1/1 -> I/1
  Current Measurement1/1 -> Fourier1/1, Current Magnitude  & Phase1/1
  connections:
  +/RConn1 -- Current Measurement1/LConn1
  Current Measurement1/RConn1 -- -/RConn1

== system SCo2/Analysis/Fault Connection in Symmetrical Components/Iaf+ ==
  I : powerlib/Electrical Sources/AC Current Source  Amplitude=A  Phase=P  Frequency=F  SampleTime=0  Measurements=None
  Zs : powerlib/Elements/Series RLC Branch  LConnTagsString=__new0  RConnTagsString=__new0  BranchType=R  Resistance=6e2  Inductance=1.0  SetiL0=off  InitialCurrent=0  Capacitance=1.0  Setx0=off  InitialVoltage=0  Measurements=None
  in_1 : PMIOPort  Port=1  Side=Left
  out_1 : PMIOPort  Port=2  Side=Right
  connections:
  I/RConn1 -- Zs/RConn1 -- out_1/RConn1
  in_1/RConn1 -- Zs/LConn1 -- I/LConn1

== system SCo2/Analysis/Fault Connection in Symmetrical Components/Iaf- ==
  I : powerlib/Electrical Sources/AC Current Source  Amplitude=A  Phase=P  Frequency=F  SampleTime=0  Measurements=None
  Zs : powerlib/Elements/Series RLC Branch  LConnTagsString=__new0  RConnTagsString=__new0  BranchType=R  Resistance=6e2  Inductance=1.0  SetiL0=off  InitialCurrent=0  Capacitance=1.0  Setx0=off  InitialVoltage=0  Measurements=None
  in_1 : PMIOPort  Port=1  Side=Left
  out_1 : PMIOPort  Port=2  Side=Right
  connections:
  in_1/RConn1 -- Zs/LConn1 -- I/LConn1
  I/RConn1 -- out_1/RConn1 -- Zs/RConn1

== system SCo2/Analysis/Fault Connection in Symmetrical Components/Iaf0 ==
  I : powerlib/Electrical Sources/AC Current Source  Amplitude=A  Phase=P  Frequency=F  SampleTime=0  Measurements=None
  Zs : powerlib/Elements/Series RLC Branch  LConnTagsString=__new0  RConnTagsString=__new0  BranchType=R  Resistance=6e2  Inductance=1.0  SetiL0=off  InitialCurrent=0  Capacitance=1.0  Setx0=off  InitialVoltage=0  Measurements=None
  in_1 : PMIOPort  Port=1  Side=Left
  out_1 : PMIOPort  Port=2  Side=Right
  connections:
  in_1/RConn1 -- Zs/LConn1 -- I/LConn1
  I/RConn1 -- Zs/RConn1 -- out_1/RConn1

== system SCo2/Analysis/Fault Connection in Symmetrical Components/Ibf+ ==
  I : powerlib/Electrical Sources/AC Current Source  Amplitude=A  Phase=P  Frequency=F  SampleTime=0  Measurements=None
  Zs : powerlib/Elements/Series RLC Branch  LConnTagsString=__new0  RConnTagsString=__new0  BranchType=R  Resistance=6e2  Inductance=1.0  SetiL0=off  InitialCurrent=0  Capacitance=1.0  Setx0=off  InitialVoltage=0  Measurements=None
  in_1 : PMIOPort  Port=1  Side=Left
  out_1 : PMIOPort  Port=2  Side=Right
  connections:
  in_1/RConn1 -- Zs/LConn1 -- I/LConn1
  out_1/RConn1 -- I/RConn1 -- Zs/RConn1

== system SCo2/Analysis/Fault Connection in Symmetrical Components/Ibf- ==
  I : powerlib/Electrical Sources/AC Current Source  Amplitude=A  Phase=P  Frequency=F  SampleTime=0  Measurements=None
  Zs : powerlib/Elements/Series RLC Branch  LConnTagsString=__new0  RConnTagsString=__new0  BranchType=R  Resistance=6e2  Inductance=1.0  SetiL0=off  InitialCurrent=0  Capacitance=1.0  Setx0=off  InitialVoltage=0  Measurements=None
  in_1 : PMIOPort  Port=1  Side=Left
  out_1 : PMIOPort  Port=2  Side=Right
  connections:
  I/RConn1 -- Zs/RConn1 -- out_1/RConn1
  in_1/RConn1 -- Zs/LConn1 -- I/LConn1

== system SCo2/Analysis/Fault Connection in Symmetrical Components/Ibf0 ==
  I : powerlib/Electrical Sources/AC Current Source  Amplitude=A  Phase=P  Frequency=F  SampleTime=0  Measurements=None
  Zs : powerlib/Elements/Series RLC Branch  LConnTagsString=__new0  RConnTagsString=__new0  BranchType=R  Resistance=6e2  Inductance=1.0  SetiL0=off  InitialCurrent=0  Capacitance=1.0  Setx0=off  InitialVoltage=0  Measurements=None
  in_1 : PMIOPort  Port=1  Side=Left
  out_1 : PMIOPort  Port=2  Side=Right
  connections:
  out_1/RConn1 -- Zs/RConn1 -- I/RConn1
  in_1/RConn1 -- Zs/LConn1 -- I/LConn1

== system SCo2/Analysis/Fault Connection in Symmetrical Components/Icf+ ==
  I : powerlib/Electrical Sources/AC Current Source  Amplitude=A  Phase=P  Frequency=F  SampleTime=0  Measurements=None
  Zs : powerlib/Elements/Series RLC Branch  LConnTagsString=__new0  RConnTagsString=__new0  BranchType=R  Resistance=6e2  Inductance=1.0  SetiL0=off  InitialCurrent=0  Capacitance=1.0  Setx0=off  InitialVoltage=0  Measurements=None
  in_1 : PMIOPort  Port=1  Side=Left
  out_1 : PMIOPort  Port=2  Side=Right
  connections:
  out_1/RConn1 -- Zs/RConn1 -- I/RConn1
  in_1/RConn1 -- Zs/LConn1 -- I/LConn1

== system SCo2/Analysis/Fault Connection in Symmetrical Components/Icf- ==
  I : powerlib/Electrical Sources/AC Current Source  Amplitude=A  Phase=P  Frequency=F  SampleTime=0  Measurements=None
  Zs : powerlib/Elements/Series RLC Branch  LConnTagsString=__new0  RConnTagsString=__new0  BranchType=R  Resistance=6e2  Inductance=1.0  SetiL0=off  InitialCurrent=0  Capacitance=1.0  Setx0=off  InitialVoltage=0  Measurements=None
  in_1 : PMIOPort  Port=1  Side=Left
  out_1 : PMIOPort  Port=2  Side=Right
  connections:
  out_1/RConn1 -- Zs/RConn1 -- I/RConn1
  in_1/RConn1 -- Zs/LConn1 -- I/LConn1

== system SCo2/Analysis/Fault Connection in Symmetrical Components/Icf0 ==
  I : powerlib/Electrical Sources/AC Current Source  Amplitude=A  Phase=P  Frequency=F  SampleTime=0  Measurements=None
  Zs : powerlib/Elements/Series RLC Branch  LConnTagsString=__new0  RConnTagsString=__new0  BranchType=R  Resistance=6e2  Inductance=1.0  SetiL0=off  InitialCurrent=0  Capacitance=1.0  Setx0=off  InitialVoltage=0  Measurements=None
  in_1 : PMIOPort  Port=1  Side=Left
  out_1 : PMIOPort  Port=2  Side=Right
  connections:
  I/RConn1 -- Zs/RConn1 -- out_1/RConn1
  in_1/RConn1 -- Zs/LConn1 -- I/LConn1

== system SCo2/Analysis/Fault Connection in Symmetrical Components/Voltage  Measurement ==
  Fourier2 : powerlib_extras/Measurements/Fourier  f1=60  n=1
  Mux3 : Mux  Inputs=2
  Voltage Measurement1 : powerlib/Measurements/Voltage Measurement  PhasorSimulation=off  OutputType=Magnitude  PSBequivalent=0
  + : PMIOPort  Port=1  Side=Left
  - : PMIOPort  Port=2  Side=Left
  V : Outport  InitialOutput=0
  wires:
  Fourier2/1 -> Mux3/1
  Fourier2/2 -> Mux3/2
  Mux3/1 -> V/1
  Voltage Measurement1/1 -> Fourier2/1
  connections:
  +/RConn1 -- Voltage Measurement1/LConn1
  -/RConn1 -- Voltage Measurement1/LConn2

== system SCo2/Analysis/Negative Sequence Network/Current  Measurement ==
  Current Measurement1 : powerlib/Measurements/Current Measurement  PhasorSimulation=off  OutputType=Magnitude  PSBequivalent=0
  Fourier1 : powerlib_extras/Measurements/Fourier  f1=60  n=1
  Mux1 : Mux  Inputs=2
  + : PMIOPort  Port=1  Side=Left
  - : PMIOPort  Port=2  Side=Right
  I : Outport  InitialOutput=0
  wires:
  Fourier1/2 -> Mux1/2
  Fourier1/1 -> Mux1/1
  Mux1/1 -> I/1
  Current Measurement1/1 -> Fourier1/1
  connections:
  +/RConn1 -- Current Measurement1/LConn1
  Current Measurement1/RConn1 -- -/RConn1

== system SCo2/Analysis/Negative Sequence Network/Iaf- ==
  I : powerlib/Electrical Sources/AC Current Source  Amplitude=A  Phase=P  Frequency=F  SampleTime=0  Measurements=None
  Zs : powerlib/Elements/Series RLC Branch  LConnTagsString=__new0  RConnTagsString=__new0  BranchType=R  Resistance=1e2  Inductance=1.0  SetiL0=off  InitialCurrent=0  Capacitance=1.0  Setx0=off  InitialVoltage=0  Measurements=None
  in_1 : PMIOPort  Port=1  Side=Left
  out_1 : PMIOPort  Port=2  Side=Right
  connections:
  Zs/RConn1 -- I/RConn1 -- out_1/RConn1
  in_1/RConn1 -- Zs/LConn1 -- I/LConn1

== system SCo2/Analysis/Negative Sequence Network/V- ==
  Fourier2 : powerlib_extras/Measurements/Fourier  f1=60  n=1
  Mux3 : Mux  Inputs=2
  Voltage Measurement1 : powerlib/Measurements/Voltage Measurement  PhasorSimulation=off  OutputType=Magnitude  PSBequivalent=0
  + : PMIOPort  Port=1  Side=Left
  - : PMIOPort  Port=2  Side=Left
  V : Outport  InitialOutput=0
  wires:
  Fourier2/1 -> Mux3/1
  Fourier2/2 -> Mux3/2
  Mux3/1 -> V/1
  Voltage Measurement1/1 -> Fourier2/1
  connections:
  +/RConn1 -- Voltage Measurement1/LConn1
  -/RConn1 -- Voltage Measurement1/LConn2

== system SCo2/Analysis/Positive Sequence Network/Current  Measurement ==
  Current Measurement1 : powerlib/Measurements/Current Measurement  PhasorSimulation=off  OutputType=Magnitude  PSBequivalent=0
  Fourier1 : powerlib_extras/Measurements/Fourier  f1=60  n=1
  Mux1 : Mux  Inputs=2
  + : PMIOPort  Port=1  Side=Left
  - : PMIOPort  Port=2  Side=Right
  I : Outport  InitialOutput=0
  wires:
  Fourier1/2 -> Mux1/2
  Fourier1/1 -> Mux1/1
  Mux1/1 -> I/1
  Current Measurement1/1 -> Fourier1/1
  connections:
  +/RConn1 -- Current Measurement1/LConn1
  Current Measurement1/RConn1 -- -/RConn1

== system SCo2/Analysis/Positive Sequence Network/Iaf+ ==
  I : powerlib/Electrical Sources/AC Current Source  Amplitude=A  Phase=P  Frequency=F  SampleTime=0  Measurements=None
  Zs : powerlib/Elements/Series RLC Branch  LConnTagsString=__new0  RConnTagsString=__new0  BranchType=R  Resistance=1e2  Inductance=1.0  SetiL0=off  InitialCurrent=0  Capacitance=1.0  Setx0=off  InitialVoltage=0  Measurements=None
  in_1 : PMIOPort  Port=1  Side=Left
  out_1 : PMIOPort  Port=2  Side=Right
  connections:
  in_1/RConn1 -- Zs/LConn1 -- I/LConn1
  I/RConn1 -- Zs/RConn1 -- out_1/RConn1

== system SCo2/Analysis/Positive Sequence Network/V+ ==
  Fourier2 : powerlib_extras/Measurements/Fourier  f1=60  n=1
  Mux3 : Mux  Inputs=2
  Voltage Measurement1 : powerlib/Measurements/Voltage Measurement  PhasorSimulation=off  OutputType=Magnitude  PSBequivalent=0
  + : PMIOPort  Port=1  Side=Left
  - : PMIOPort  Port=2  Side=Left
  V : Outport  InitialOutput=0
  wires:
  Fourier2/1 -> Mux3/1
  Fourier2/2 -> Mux3/2
  Mux3/1 -> V/1
  Voltage Measurement1/1 -> Fourier2/1
  connections:
  +/RConn1 -- Voltage Measurement1/LConn1
  -/RConn1 -- Voltage Measurement1/LConn2

== system SCo2/Analysis/Zero Sequence Network/Current  Measurement ==
  Current Measurement1 : powerlib/Measurements/Current Measurement  PhasorSimulation=off  OutputType=Magnitude  PSBequivalent=0
  Fourier1 : powerlib_extras/Measurements/Fourier  f1=60  n=1
  Mux1 : Mux  Inputs=2
  + : PMIOPort  Port=1  Side=Left
  - : PMIOPort  Port=2  Side=Right
  I : Outport  InitialOutput=0
  wires:
  Fourier1/2 -> Mux1/2
  Fourier1/1 -> Mux1/1
  Mux1/1 -> I/1
  Current Measurement1/1 -> Fourier1/1
  connections:
  +/RConn1 -- Current Measurement1/LConn1
  Current Measurement1/RConn1 -- -/RConn1

== system SCo2/Analysis/Zero Sequence Network/Iaf0 ==
  I : powerlib/Electrical Sources/AC Current Source  Amplitude=A  Phase=P  Frequency=F  SampleTime=0  Measurements=None
  Zs : powerlib/Elements/Series RLC Branch  LConnTagsString=__new0  RConnTagsString=__new0  BranchType=R  Resistance=1e2  Inductance=1.0  SetiL0=off  InitialCurrent=0  Capacitance=1.0  Setx0=off  InitialVoltage=0  Measurements=None
  in_1 : PMIOPort  Port=1  Side=Left
  out_1 : PMIOPort  Port=2  Side=Right
  connections:
  out_1/RConn1 -- I/RConn1 -- Zs/RConn1
  in_1/RConn1 -- Zs/LConn1 -- I/LConn1

== system SCo2/Analysis/Zero Sequence Network/V0 ==
  Fourier2 : powerlib_extras/Measurements/Fourier  f1=60  n=1
  Mux3 : Mux  Inputs=2
  Voltage Measurement1 : powerlib/Measurements/Voltage Measurement  PhasorSimulation=off  OutputType=Magnitude  PSBequivalent=0
  + : PMIOPort  Port=1  Side=Left
  - : PMIOPort  Port=2  Side=Left
  V : Outport  InitialOutput=0
  wires:
  Fourier2/1 -> Mux3/1
  Fourier2/2 -> Mux3/2
  Mux3/1 -> V/1
  Voltage Measurement1/1 -> Fourier2/1
  connections:
  +/RConn1 -- Voltage Measurement1/LConn1
  -/RConn1 -- Voltage Measurement1/LConn2

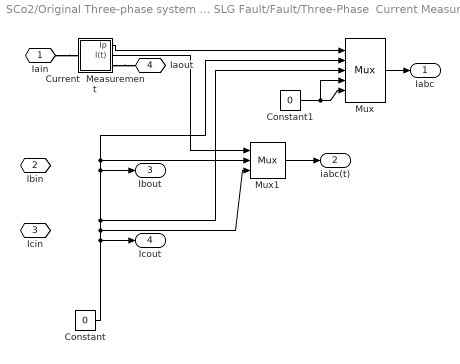
== system SCo2/Original Three-phase system with a SLG Fault/Fault/Three-Phase  Current Measuremnet ==
  Constant : Constant  Value=0
  Constant1 : Constant  Value=0
  Current  Measurement : Subsystem
  Mux : Mux  Inputs=5
  Mux1 : Mux  Inputs=3
  Iain : PMIOPort  Port=1  Side=Left
  Ibin : PMIOPort  Port=2  Side=Left
  Icin : PMIOPort  Port=3  Side=Left
  Iaout : PMIOPort  Port=4  Side=Right
  Iabc : Outport  InitialOutput=0
  iabc(t) : Outport  Port=2  InitialOutput=0
  Ibout : Outport  Port=3  InitialOutput=0
  Icout : Outport  Port=4  InitialOutput=0
  wires:
  Mux/1 -> Iabc/1
  Current  Measurement/1(Ip) -> Mux/1
  Mux1/1 -> iabc(t)/1
  Current  Measurement/2(I(t)) -> Mux1/1
  Constant/1 -> Mux/2, Mux1/2, Ibout/1, Mux/3, Mux1/3, Icout/1
  Constant1/1 -> Mux/5, Mux/4
  connections:
  Iain/RConn1 -- Current  Measurement/LConn1
  Current  Measurement/RConn1 -- Iaout/RConn1

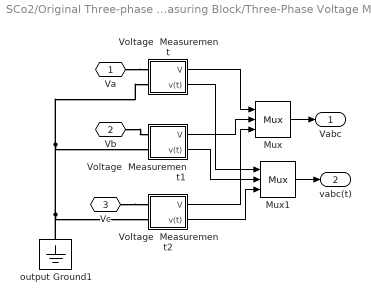
== system SCo2/Original Three-phase system with a SLG Fault/Measuring Block/Three-Phase Voltage Measurements ==
  Mux : Mux  Inputs=3
  Mux1 : Mux  Inputs=3
  Voltage  Measurement : Subsystem
  Voltage  Measurement1 : Subsystem
  Voltage  Measurement2 : Subsystem
  output Ground1 : powerlib/Elements/Ground  LConnTagsString=a
  Va : PMIOPort  Port=1  Side=Left
  Vb : PMIOPort  Port=2  Side=Left
  Vc : PMIOPort  Port=3  Side=Left
  Vabc : Outport  InitialOutput=0
  vabc(t) : Outport  Port=2  InitialOutput=0
  wires:
  Voltage  Measurement/1(V) -> Mux/1
  Voltage  Measurement1/1(V) -> Mux/2
  Voltage  Measurement2/1(V) -> Mux/3
  Voltage  Measurement/2(v(t)) -> Mux1/1
  Voltage  Measurement1/2(v(t)) -> Mux1/2
  Voltage  Measurement2/2(v(t)) -> Mux1/3
  Mux/1 -> Vabc/1
  Mux1/1 -> vabc(t)/1
  connections:
  output Ground1/LConn1 -- Voltage  Measurement/LConn2 -- Voltage  Measurement1/LConn2 -- Voltage  Measurement2/LConn2
  Va/RConn1 -- Voltage  Measurement/LConn1
  Vb/RConn1 -- Voltage  Measurement1/LConn1
  Vc/RConn1 -- Voltage  Measurement2/LConn1

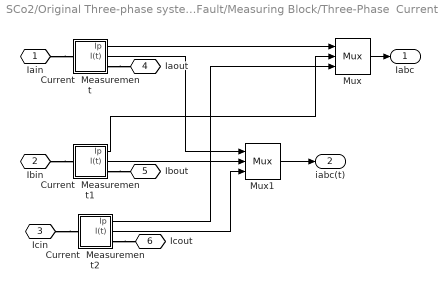
== system SCo2/Original Three-phase system with a SLG Fault/Measuring Block/Three-Phase  Current Measurements ==
  Current  Measurement : Subsystem
  Current  Measurement1 : Subsystem
  Current  Measurement2 : Subsystem
  Mux : Mux  Inputs=3
  Mux1 : Mux  Inputs=3
  Iain : PMIOPort  Port=1  Side=Left
  Ibin : PMIOPort  Port=2  Side=Left
  Icin : PMIOPort  Port=3  Side=Left
  Iaout : PMIOPort  Port=4  Side=Right
  Ibout : PMIOPort  Port=5  Side=Right
  Icout : PMIOPort  Port=6  Side=Right
  Iabc : Outport  InitialOutput=0
  iabc(t) : Outport  Port=2  InitialOutput=0
  wires:
  Mux/1 -> Iabc/1
  Current  Measurement/1(Ip) -> Mux/1
  Current  Measurement1/1(Ip) -> Mux/2
  Current  Measurement2/1(Ip) -> Mux/3
  Mux1/1 -> iabc(t)/1
  Current  Measurement/2(I(t)) -> Mux1/1
  Current  Measurement1/2(I(t)) -> Mux1/2
  Current  Measurement2/2(I(t)) -> Mux1/3
  connections:
  Iain/RConn1 -- Current  Measurement/LConn1
  Current  Measurement/RConn1 -- Iaout/RConn1
  Ibin/RConn1 -- Current  Measurement1/LConn1
  Current  Measurement1/RConn1 -- Ibout/RConn1
  Icin/RConn1 -- Current  Measurement2/LConn1
  Current  Measurement2/RConn1 -- Icout/RConn1

== system SCo2/Original Three-phase system with a SLG Fault/Fault/Three-Phase  Current Measuremnet/Current  Measurement ==
  Current Measurement1 : powerlib/Measurements/Current Measurement  PhasorSimulation=off  OutputType=Magnitude  PSBequivalent=0
  Fourier1 : powerlib_extras/Measurements/Fourier  f1=60  n=1
  Mux1 : Mux  Inputs=2
  + : PMIOPort  Port=1  Side=Left
  - : PMIOPort  Port=2  Side=Right
  Ip : Outport  InitialOutput=0
  I(t) : Outport  Port=2  InitialOutput=0
  wires:
  Fourier1/2 -> Mux1/2
  Fourier1/1 -> Mux1/1
  Mux1/1 -> Ip/1
  Current Measurement1/1 -> I(t)/1, Fourier1/1
  connections:
  +/RConn1 -- Current Measurement1/LConn1
  Current Measurement1/RConn1 -- -/RConn1

== system SCo2/Original Three-phase system with a SLG Fault/Measuring Block/Three-Phase Voltage Measurements/Voltage  Measurement ==
  Fourier2 : powerlib_extras/Measurements/Fourier  f1=60  n=1
  Mux3 : Mux  Inputs=2
  Voltage Measurement1 : powerlib/Measurements/Voltage Measurement  PhasorSimulation=off  OutputType=Magnitude  PSBequivalent=0
  + : PMIOPort  Port=1  Side=Left
  - : PMIOPort  Port=2  Side=Left
  V : Outport  InitialOutput=0
  v(t) : Outport  Port=2  InitialOutput=0
  wires:
  Fourier2/1 -> Mux3/1
  Fourier2/2 -> Mux3/2
  Mux3/1 -> V/1
  Voltage Measurement1/1 -> Fourier2/1, v(t)/1
  connections:
  +/RConn1 -- Voltage Measurement1/LConn1
  -/RConn1 -- Voltage Measurement1/LConn2

== system SCo2/Original Three-phase system with a SLG Fault/Measuring Block/Three-Phase Voltage Measurements/Voltage  Measurement1 ==
  Fourier2 : powerlib_extras/Measurements/Fourier  f1=60  n=1
  Mux3 : Mux  Inputs=2
  Voltage Measurement1 : powerlib/Measurements/Voltage Measurement  PhasorSimulation=off  OutputType=Magnitude  PSBequivalent=0
  + : PMIOPort  Port=1  Side=Left
  - : PMIOPort  Port=2  Side=Left
  V : Outport  InitialOutput=0
  v(t) : Outport  Port=2  InitialOutput=0
  wires:
  Mux3/1 -> V/1
  Fourier2/2 -> Mux3/2
  Fourier2/1 -> Mux3/1
  Voltage Measurement1/1 -> v(t)/1, Fourier2/1
  connections:
  -/RConn1 -- Voltage Measurement1/LConn2
  +/RConn1 -- Voltage Measurement1/LConn1

== system SCo2/Original Three-phase system with a SLG Fault/Measuring Block/Three-Phase Voltage Measurements/Voltage  Measurement2 ==
  Fourier2 : powerlib_extras/Measurements/Fourier  f1=60  n=1
  Mux3 : Mux  Inputs=2
  Voltage Measurement1 : powerlib/Measurements/Voltage Measurement  PhasorSimulation=off  OutputType=Magnitude  PSBequivalent=0
  + : PMIOPort  Port=1  Side=Left
  - : PMIOPort  Port=2  Side=Left
  V : Outport  InitialOutput=0
  v(t) : Outport  Port=2  InitialOutput=0
  wires:
  Fourier2/1 -> Mux3/1
  Fourier2/2 -> Mux3/2
  Mux3/1 -> V/1
  Voltage Measurement1/1 -> Fourier2/1, v(t)/1
  connections:
  +/RConn1 -- Voltage Measurement1/LConn1
  -/RConn1 -- Voltage Measurement1/LConn2

== system SCo2/Original Three-phase system with a SLG Fault/Measuring Block/Three-Phase  Current Measurements/Current  Measurement ==
  Current Measurement1 : powerlib/Measurements/Current Measurement  PhasorSimulation=off  OutputType=Magnitude  PSBequivalent=0
  Fourier1 : powerlib_extras/Measurements/Fourier  f1=60  n=1
  Mux1 : Mux  Inputs=2
  + : PMIOPort  Port=1  Side=Left
  - : PMIOPort  Port=2  Side=Right
  Ip : Outport  InitialOutput=0
  I(t) : Outport  Port=2  InitialOutput=0
  wires:
  Fourier1/2 -> Mux1/2
  Fourier1/1 -> Mux1/1
  Mux1/1 -> Ip/1
  Current Measurement1/1 -> I(t)/1, Fourier1/1
  connections:
  +/RConn1 -- Current Measurement1/LConn1
  Current Measurement1/RConn1 -- -/RConn1

== system SCo2/Original Three-phase system with a SLG Fault/Measuring Block/Three-Phase  Current Measurements/Current  Measurement1 ==
  Current Measurement1 : powerlib/Measurements/Current Measurement  PhasorSimulation=off  OutputType=Magnitude  PSBequivalent=0
  Fourier1 : powerlib_extras/Measurements/Fourier  f1=60  n=1
  Mux1 : Mux  Inputs=2
  + : PMIOPort  Port=1  Side=Left
  - : PMIOPort  Port=2  Side=Right
  Ip : Outport  InitialOutput=0
  I(t) : Outport  Port=2  InitialOutput=0
  wires:
  Mux1/1 -> Ip/1
  Fourier1/1 -> Mux1/1
  Fourier1/2 -> Mux1/2
  Current Measurement1/1 -> Fourier1/1, I(t)/1
  connections:
  Current Measurement1/RConn1 -- -/RConn1
  +/RConn1 -- Current Measurement1/LConn1
